simulink model "arcsensors"  (R2025b)
settings: Solver=ode4  StartTime=0.0  StopTime=10.0  FixedStep=0.002  RelTol=1e-3
undefined symbols (not defined in the file or in its folder): fractalcoef
libraries: mspfiltlib x1, robotcorelib x1, simulink x1, sensorgpslib x1, mspsensorlib x1, matrix_library x1
settings Model: Creator=ryanb  LastModifiedBy=ryanb
settings SolverCC: ConcurrentTasks=on

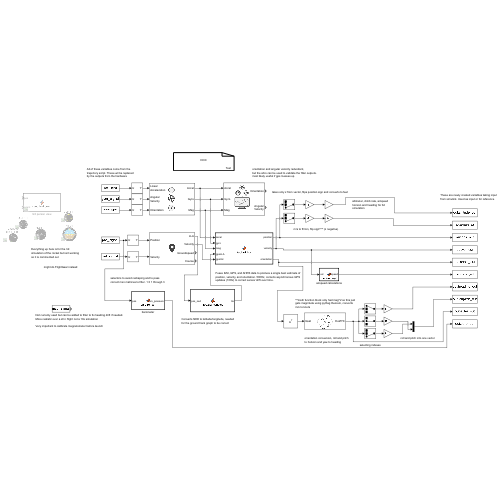
[thumbnail: Simulink's stored preview of the top-level diagram]
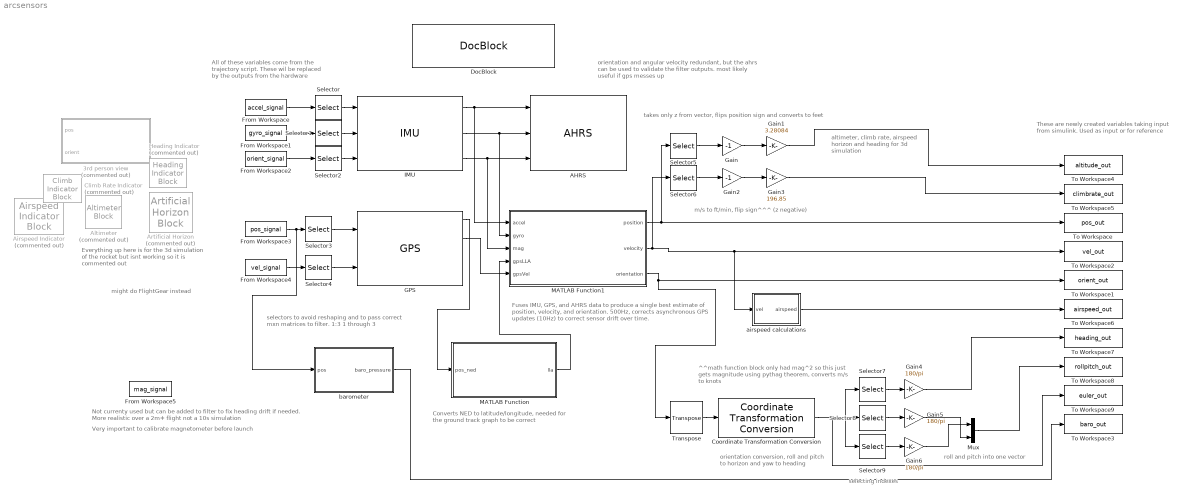
== system arcsensors ==
  note: Converts NED to latitude/longitude, needed
      | for the ground track graph to be correct
  note: selecting indexes
  note: These are newly created variables taking input
      | from simulink. Used as input or for reference
  note: All of these variables come from the
      | trajectory script. These wil be replaced
      | by the outputs from the hardware
  note: Very important to calibrate magnetometer before launch
  note: roll and pitch into one vector
  note: might do FlightGear instead
  note: Everything up here is for the 3d
      | simulation of the rocket but isnt working
      | so it is commented out
  note: altimeter, climb rate, airspeed
      | horizon and heading for 3d
      | simulation
  note: orientation conversion, roll and pitch
      | to horizon and yaw to heading
  note: ^^math function block only had mag^2 so this just
      | gets magnitude using pythag theorem, converts
      | m/s to knots
  note: m/s to ft/min, flip sign^^^ (z negative)
  note: takes only z from vector, flips position sign and converts to feet
  note: orientation and angular velocity redundant,
      | but the ahrs can be used to validate the filter outputs.
      | most likely useful if gps messes up
  note: selectors to avoid reshaping and to pass
      | correct mxn matrices to filter. 1:3 1 through 3
  note: Not currenty used but can be added to filter to fix heading drift if needed.
      | More realistic over a 2m+ flight not a 10s simulation
  note: Fuses IMU, GPS, and AHRS data to produce a single best estimate of
      | position, velocity, and orientation. 500Hz, corrects asynchronous GPS
      | updates (10Hz) to correct sensor drift over time.
  3rd person view : MATLAB Function  Commented=on  TreatAsAtomicUnit=on
  AHRS : mspfiltlib/AHRS  DispRefFrame=NED  DecimationFactor=1  InitialProcessNoise=ahrsfilter.defaultProcessNoise  OrientationFormat=quaternion  SimulateUsing=Interpreted execution  AccelerometerNoise=0.0001924722  GyroscopeNoise=9.1385e-5  MagnetometerNoise=0.1  GyroscopeDriftNoise=3.0462e-13  LinearAccelerationNoise=0.0096236100000000012  MagneticDisturbanceNoise=0.5  LinearAccelerationDecayFactor=0.5  MagneticDisturbanceDecayFactor=0.5  ExpectedMagneticFieldStrength=50
  Airspeed Indicator : AirspeedIndicatorBlock  Commented=on  ScaleMin=20  ScaleMax=600
  Altimeter : AltimeterBlock  Commented=on
  Artificial Horizon : ArtificialHorizonBlock  Commented=on
  Climb Rate Indicator : ClimbIndicatorBlock  Commented=on  ScaleMax=10000
  Coordinate Transformation Conversion : robotcorelib/Coordinate Transformation Conversion  InputRepresentation=Quaternion  InputEulerSequence=ZYX  ShowTrVecInputPort=on  OutputRepresentation=Euler Angles  OutputEulerSequence=ZYX  ShowTrVecOutputPort=on  SimulateUsing=Interpreted execution
      settings: LibrarySourceBlock=navlib/Utilities/Coordinate Transformation Conversion
  DocBlock : simulink/Model-Wide Utilities/DocBlock  DocumentType=Text
      content=|
      | MATLAB Simulink Project
      | ARCUIA
      | Ryan Breen
      |
      | Sensors
      | accelerometer acceleration m/s^2
      | gyro rad/s (convert from deg/s)
      | (x, y, z for both) + other parameters if necessary
      | - Outputs acceleration & gyro vectors
      | Clock included for timestamp
      |
      | magnometer microtesla (mu T)
      | Input mag vector (x, y, z), calibration
      | Output mag vector & timestamp if needed
      | - Finds absolute yaw (heading) corrects altitude
      |
      | GPS/GNSS reciever position m/s (ENU/NED convert)
      | Input GNSS data stream, antenna status, configuration
      | Output (x,y,z lat/long), velocity, fix status & timestamp
      |
      | PPS/1PPS pulse/s
      | gives pulses per second for timestamp alignemnt
      | Input hardware interrupt pin
      | Output precise timestamp events and sunc signals from other sensors
      | Syncrhonize hardware from asynchronized sensors
      |
      | Barometer pressure Pa
      | converted to altitude in m
      | Input raw pressure reading, temp
      | Output altitude, barometric pressure (Pa) and a timestamp
      |
      | Pitot/Airspeed sensor (Pa -> airspeed in m/s)
      | Inputs pitot pressure, static pressure, temp
      | Outputs calibrated airspeed in and a timestamp
      | Function to convert the barometer data into a target airspeed
      | Navigation and Control
      |
      | - At this point we have altitude, timestamps, airspeed,
      | direction of acceleration, yaw, pressure, and location
      |
      | - We still need temp & video. Along with that, there are a
      | couple of other sensors that could be added:
      |
      | External Heading Source (high precision position, m, rad)
      | Wheel Encoders or Speed Sensors (velocity, timestamps)
      | External triggers to coordinate asynchronous events
      | ^^Not included because I do not know if they are applicable
      |
      | Important Notes:
      | -always include timestamp with each sensor output as a baseline
      | -make sure you have the correct units, sometimes you have
      | to convert, typically degrees to radians or NED vs ENU for the gps
      | -conversions can be done with the matlab function block and you code it
      |
      | Final Notes:
      | -Set sample time, removed clock, just put dt as a variable
      | -Going to add 3d model
      | -Graphs look good but currently have no noise so I need to
      | see how it is with hardware and see if they still look good
      | -AHRS filter redundant, but can validate the main filter if gps
      | messes up
  From Workspace : FromWorkspace  VariableName=accel_signal  SampleTime=1/500  OutputAfterFinalValue=Holding final value
  From Workspace1 : FromWorkspace  VariableName=gyro_signal  SampleTime=1/500  OutputAfterFinalValue=Holding final value
  From Workspace2 : FromWorkspace  VariableName=orient_signal  SampleTime=1/500  OutputAfterFinalValue=Holding final value
  From Workspace3 : FromWorkspace  VariableName=pos_signal  SampleTime=1/500  OutputAfterFinalValue=Holding final value
  From Workspace4 : FromWorkspace  VariableName=vel_signal  SampleTime=1/500  OutputAfterFinalValue=Holding final value
  From Workspace5 : FromWorkspace  VariableName=mag_signal  SampleTime=1/500  OutputAfterFinalValue=Holding final value
  GPS : sensorgpslib/GPS  DispRefFrame=NED  PositionInputFormat=Local  ReferenceLocation=[ 0, 0, 0 ]  HorizontalPositionAccuracy=1.6  VerticalPositionAccuracy=3  VelocityAccuracy=0.1  DecayFactor=0.999  SeedDouble=67  SimulateUsing=Code generation
      settings: LibrarySourceBlock=mspsensorlib/GPS
  Gain : Gain  Gain=-1
  Gain1 : Gain  Gain=3.28084
  Gain2 : Gain  Gain=-1
  Gain3 : Gain  Gain=196.85
  Gain4 : Gain  Gain=180/pi
  Gain5 : Gain  Gain=180/pi
  Gain6 : Gain  Gain=180/pi
  Heading Indicator : HeadingIndicatorBlock  Commented=on
  IMU : mspsensorlib/IMU  DispRefFrame=NED  TemperaturePort=off  Temperature=25  MagneticFieldPort=off  MagneticFieldNED=[ 27.5550, -2.4169, -16.0849 ]  MagneticFieldENU=[ -2.4169, 27.5550, 16.0849 ]  SeedDouble=67  SimulateUsing=Interpreted execution  AccelParamsMeasurementRange=Inf  AccelParamsResolution=0  AccelParamsConstantBias=[ 0, 0, 0 ]  AccelParamsAxesMisalignment=[ 100, 0, 0; 0, 100, 0; 0, 0, 100 ]  AccelParamsNoiseDensity=[ 0, 0, 0 ]  AccelParamsBiasInstability=[ 0, 0, 0 ]  AccelParamsBiasInstabilityNumerator=fractalcoef().Numerator  AccelParamsBiasInstabilityDenominator=fractalcoef().Denominator  AccelParamsRandomWalk=[ 0, 0, 0 ]  AccelParamsNoiseType=double-sided  AccelParamsTemperatureBias=[ 0, 0, 0 ]  AccelParamsTemperatureScaleFactor=[ 0, 0, 0 ]  GyroParamsMeasurementRange=Inf  GyroParamsResolution=0  GyroParamsConstantBias=[ 0, 0, 0 ]  GyroParamsAxesMisalignment=[ 100, 0, 0; 0, 100, 0; 0, 0, 100 ]  GyroParamsAccelerationBias=[ 0, 0, 0 ]  GyroParamsNoiseDensity=[ 0, 0, 0 ]  GyroParamsBiasInstability=[ 0, 0, 0 ]  GyroParamsBiasInstabilityNumerator=fractalcoef().Numerator  GyroParamsBiasInstabilityDenominator=fractalcoef().Denominator  GyroParamsRandomWalk=[ 0, 0, 0 ]  GyroParamsNoiseType=double-sided  GyroParamsTemperatureBias=[ 0, 0, 0 ]  GyroParamsTemperatureScaleFactor=[ 0, 0, 0 ]  MagParamsMeasurementRange=Inf  MagParamsResolution=0  MagParamsConstantBias=[ 0, 0, 0 ]  MagParamsAxesMisalignment=[ 100, 0, 0; 0, 100, 0; 0, 0, 100 ]  MagParamsNoiseDensity=[ 0, 0, 0 ]  MagParamsBiasInstability=[ 0, 0, 0 ]  MagParamsBiasInstabilityNumerator=fractalcoef().Numerator  MagParamsBiasInstabilityDenominator=fractalcoef().Denominator  MagParamsRandomWalk=[ 0, 0, 0 ]  MagParamsNoiseType=double-sided  MagParamsTemperatureBias=[ 0, 0, 0 ]  MagParamsTemperatureScaleFactor=[ 0, 0, 0 ]
  MATLAB Function : MATLAB Function  TreatAsAtomicUnit=on
  MATLAB Function1 : MATLAB Function  TreatAsAtomicUnit=on
  Mux : Mux  Inputs=2
  Selector{,1,3..4} (4 alike) : Selector  NumberOfDimensions=2  InputPortWidth=3  IndexOptions=Index vector (dialog),Index vector (dialog)  Indices=1,1:3  OutputSizes=1,1
  Selector2 : Selector  NumberOfDimensions=2  InputPortWidth=3  IndexOptions=Index vector (dialog),Index vector (dialog)  Indices=1,1:4  OutputSizes=1,1
  Selector5 : Selector  InputPortWidth=3  IndexOptions=Index vector (dialog)  Indices=3  OutputSizes=1
  Selector6 : Selector  InputPortWidth=3  IndexOptions=Index vector (dialog)  Indices=3  OutputSizes=1
  Selector7 : Selector  InputPortWidth=3  IndexOptions=Index vector (dialog)  Indices=1  OutputSizes=1
  Selector8 : Selector  InputPortWidth=3  IndexOptions=Index vector (dialog)  Indices=2  OutputSizes=1
  Selector9 : Selector  InputPortWidth=3  IndexOptions=Index vector (dialog)  Indices=3  OutputSizes=1
  To Workspace : ToWorkspace  VariableName=pos_out  SaveFormat=Timeseries  SampleTime=-1
      settings: Save2DSignal=2-D array (concatenate along first dimension)
  To Workspace1 : ToWorkspace  VariableName=orient_out  SaveFormat=Timeseries  SampleTime=-1
      settings: Save2DSignal=2-D array (concatenate along first dimension)
  To Workspace2 : ToWorkspace  VariableName=vel_out  SaveFormat=Timeseries  SampleTime=-1
      settings: Save2DSignal=2-D array (concatenate along first dimension)
  To Workspace3 : ToWorkspace  VariableName=baro_out  SaveFormat=Timeseries  SampleTime=-1
  To Workspace4 : ToWorkspace  VariableName=altitude_out  SaveFormat=Timeseries  SampleTime=-1
  To Workspace5 : ToWorkspace  VariableName=climbrate_out  SaveFormat=Timeseries  SampleTime=-1
  To Workspace6 : ToWorkspace  VariableName=airspeed_out  SaveFormat=Timeseries  SampleTime=-1
  To Workspace7 : ToWorkspace  VariableName=heading_out  SaveFormat=Timeseries  SampleTime=-1
  To Workspace8 : ToWorkspace  VariableName=rollpitch_out  SaveFormat=Timeseries  SampleTime=-1
  To Workspace9 : ToWorkspace  VariableName=euler_out  SaveFormat=Timeseries  SampleTime=-1
  Transpose : matrix_library/Transpose
  airspeed calculations : MATLAB Function  TreatAsAtomicUnit=on
  barometer : MATLAB Function  TreatAsAtomicUnit=on
  wires:
  IMU/2 -> MATLAB Function1/2(gyro), AHRS/2
  IMU/1 -> AHRS/1, MATLAB Function1/1(accel)
  IMU/3 -> AHRS/3, MATLAB Function1/3(mag)
  GPS/1 -> MATLAB Function/1(pos_ned)
  GPS/2 -> MATLAB Function1/5(gpsVel)
  From Workspace/1 -> Selector/1
  From Workspace1/1 -> Selector1/1
  From Workspace2/1 -> Selector2/1
  From Workspace3/1 -> barometer/1(pos), Selector3/1
  From Workspace4/1 -> Selector4/1
  MATLAB Function1/1(position) -> To Workspace/1, Selector5/1
  MATLAB Function1/3(orientation) -> Transpose/1, To Workspace1/1
  Selector4/1 -> GPS/2
  Selector3/1 -> GPS/1
  Selector/1 -> IMU/1
  Selector1/1 -> IMU/2
  Selector2/1 -> IMU/3
  Gain/1 -> Gain1/1
  Selector5/1 -> Gain/1
  MATLAB Function1/2(velocity) -> airspeed calculations/1(vel), To Workspace2/1, Selector6/1
  Selector6/1 -> Gain2/1
  Gain2/1 -> Gain3/1
  Coordinate Transformation Conversion/1 -> To Workspace9/1, Selector9/1, Selector7/1, Selector8/1
  Selector9/1 -> Gain6/1
  Selector8/1 -> Gain5/1
  Selector7/1 -> Gain4/1
  Gain5/1 -> Mux/2
  Gain6/1 -> Mux/1
  Transpose/1 -> Coordinate Transformation Conversion/1
  Gain1/1 -> To Workspace4/1
  Gain3/1 -> To Workspace5/1
  airspeed calculations/1(airspeed) -> To Workspace6/1
  Mux/1 -> To Workspace8/1
  Gain4/1 -> To Workspace7/1
  barometer/1(baro_pressure) -> To Workspace3/1
  MATLAB Function/1(lla) -> MATLAB Function1/4(gpsLLA)

== matlab function arcsensors/MATLAB Function1 ==
  data: accel input; position output; gyro input; mag input; gpsLLA input; gpsVel input; velocity output; orientation output
function [position, velocity, orientation] = fusionFilter(accel, gyro, mag, gpsLLA, gpsVel)
    % 1. Explicitly define outputs for the Coder
    position    = zeros(1, 3);
    velocity    = zeros(1, 3);
    orientation = zeros(1, 4);

    persistent filter initialized gpsCounter
    
    dt = 1/500; 

    if isempty(initialized)
        filter = insfilterAsync;
        filter.ReferenceLocation = [0 0 0];
        
        % Process Noise
        filter.AccelerometerBiasNoise = 1e-4;
        filter.GyroscopeBiasNoise     = 1e-9;
        
        % Initial State (R2025 Mapping)
        filter.State(1:4)   = [1 0 0 0]; % Quat
        filter.State(8:10)  = [0 0 0];    % Position
        filter.State(11:13) = [0 0 0];   % Velocity
        
        gpsCounter  = 0;
        initialized = true;
    end

    % 2. Fix the "Expected 3 columns" error
    % We grab the first 3 elements and force them into a 1x3 row vector
    curAccel = reshape(accel(1:3), 1, 3); 
    curGyro  = reshape(gyro(1:3), 1, 3);
    curMag   = reshape(mag(1:3), 1, 3);
    
    % Prediction
    predict(filter, dt);

    % Covariances
    accelCov  = diag([0.0012 0.0012 0.0012]);
    gyroCov   = diag([1e-5 1e-5 1e-5]);
    magCov    = diag([0.1 0.1 0.1]);

    % 3. Fuse data (Passing 1x3 row vectors as required)
    fuseaccel(filter, curAccel, accelCov);
    fusegyro(filter, curGyro, gyroCov);
    fusemag(filter, curMag, magCov);

    % GPS Correction at 10Hz
    gpsCounter = gpsCounter + 1;
    if gpsCounter >= 50
        % Force GPS inputs to 1x3 row vectors
        curGpsLLA = reshape(gpsLLA(1:3), 1, 3);
        curGpsVel = reshape(gpsVel(1:3), 1, 3);
        
        gpsPosCov = diag([1.6 1.6 3].^2);
        gpsVelCov = diag([0.1 0.1 0.1].^2);
        
        fusegps(filter, curGpsLLA, gpsPosCov, curGpsVel, gpsVelCov);
        gpsCounter = 0;
    end

    % 4. Fix the "quaternion does not have property w" error
    [p, q, v] = pose(filter);
    
    position    = reshape(p, 1, 3);
    velocity    = reshape(v, 1, 3);
    
    % Use 'compact' to turn the quaternion object into a [w x y z] array
    orientation = compact(q); 
end

== matlab function arcsensors/airspeed calculations ==
  data: vel input; airspeed output
function airspeed = calcAirspeed(vel)
airspeed = sqrt(vel(1)^2 +vel(2)^2 + vel(3)^2) * 1.944;

== matlab function arcsensors/3rd person view ==
  data: pos input; orient input
function visualizeRocket(pos, orient)
% Declare extrinsic functions for MATLAB Graphics
coder.extrinsic('figure', 'gcf', 'gca', 'plot3', 'hold', 'grid', 'xlabel', ...
                'ylabel', 'zlabel', 'drawnow', 'set', 'view', 'axis', ...
                'patch', 'surface', 'title', 'isgraphics', 'clf');

persistent hFig hAxes hRocket hTrail trailData stepCount

% 1. Immediate Dummy Assignment
% This is the "Magic Fix" for the Coder error.
if isempty(stepCount)
    stepCount = 0;
    hFig = 0;   % Give it a numeric value so it is "assigned"
    hAxes = 0;
    hRocket = 0;
    hTrail = 0;
    trailData = zeros(5005, 3); 
end

% 2. Check if we need to (re)initialize the window
% Since hFig is now guaranteed to be '0' or a 'Handle', this is safe.
doInit = false;
if hFig == 0
    doInit = true;
elseif ~isgraphics(hFig)
    doInit = true;
end

if doInit
    % Create the figure window
    hFig = figure('Name', 'Rocket 3D Mission Display', 'Color', 'w');
    hAxes = gca;
    hold(hAxes, 'on');
    grid(hAxes, 'on');
    
    % Frame Setup (NED)
    xlabel(hAxes, 'North (m)');
    ylabel(hAxes, 'East (m)');
    zlabel(hAxes, 'Altitude (m)'); 
    title(hAxes, 'Real-Time Sensor Fusion Trajectory');

    % Create a Ground Plane
    [G_X, G_Y] = meshgrid(-100:20:100, -100:20:100);
    G_Z = zeros(size(G_X));
    surface(hAxes, G_X, G_Y, G_Z, 'FaceAlpha', 0.1, 'EdgeColor', [0.5 0.5 0.5]);

    % Initialize graphics objects
    hTrail = plot3(hAxes, 0, 0, 0, 'b-', 'LineWidth', 1.5);
    hRocket = plot3(hAxes, 0, 0, 0, 'ro', 'MarkerFaceColor', 'r', 'MarkerSize', 8);
    
    view(hAxes, 45, 30);
    axis(hAxes, 'equal');
end

% 3. Update Logic (Runs every step at 500Hz)
stepCount = stepCount + 1;

% NED to Altitude (Down is negative, so flip it)
N = pos(1);
E = pos(2);
Alt = -pos(3); 

% Update Trail Buffer
if stepCount <= 5000
    trailData(stepCount, :) = [N, E, Alt];
end

% 4. Visual Update (Throttled to ~25Hz for performance)
if mod(stepCount, 20) == 0
    % Update the line and point
    set(hTrail, 'XData', trailData(1:stepCount, 1), ...
                'YData', trailData(1:stepCount, 2), ...
                'ZData', trailData(1:stepCount, 3));
    set(hRocket, 'XData', N, 'YData', E, 'ZData', Alt);
    
    % Chase Camera: Stay 20m back, 10m up
    set(hAxes, 'CameraPosition', [N-20, E-20, Alt+10], ...
               'CameraTarget',   [N, E, Alt]);
    
    % Adjust axis limits so the rocket doesn't fly off screen
    axis(hAxes, [N-50 N+50 E-50 E+50 0 max(100, Alt+50)]);
    
    % Force the update
    drawnow('limitrate');
end

== matlab function arcsensors/barometer ==
  data: pos input; baro_pressure output
function baro_pressure = baroSensor(pos)
    % Barometer sensor model — outputs pressure in Pa
    % Input:  pos [N E D] in meters
    % Output: noisy barometric pressure in Pa

    baro_pressure = 0;

    coder.extrinsic('atmoscoesa');

    % NED Down -> geometric altitude
    true_alt = -pos(3);

    % Standard atmosphere: altitude -> pressure
    P = 0;
    [~, ~, P, ~] = atmoscoesa(true_alt);

    % MEMS barometer noise (BMP388-class sensor)
    noise_std = 1.5;  % Pa
    baro_pressure = P + noise_std * randn;
end

== matlab function arcsensors/MATLAB Function ==
  data: pos_ned input; lla output
function lla = ned2lla_convert(pos_ned)
    lla = zeros(1, 3);
    coder.extrinsic('ned2lla');
    
    pos = reshape(pos_ned(1:3), 1, 3);
    ref = [0 0 0];  % matches filter.ReferenceLocation
    
    lla = ned2lla(pos, ref, 'ellipsoid');
end
